simulink model "scdairframe_reference"  (Simulink 7.6)
settings: Solver=ode45  SolverMode=SingleTasking  StartTime=0.0  StopTime=10.0  RelTol=1e-3  AbsTol=1e-6
model workspace (MATLAB code in the model file):
  | scd_aero_guid_dat
values from neighbouring files (symbols this model uses):
  h_ini = 10000/m2ft    (= 3047.99990246)    [scd_aero_guid_dat.m]
  Thrust = 10e3    (= 10000)    [scd_aero_guid_dat.m]
libraries: aerospace x1
settings Model: Creator=The MathWorks Inc.  ExtModeTrigMode=oneshot  ExtModeArmWhenConnect=off  ExtModeAutoUpdateStatusClock=off
settings DataIOCC: LimitDataPoints=off  SaveOutput=off  SignalLogging=off  SaveTime=off  SignalLoggingName=sigsOut
settings OptimizationCC: BlockReduction=off  BooleanDataType=off  InlineParams=on  InlineInvariantSignals=on  InitFltsAndDblsToZero=on
settings DebuggingCC: SaveWithParameterizedLinksMsg=none  CheckExecutionContextPreStartOutputMsg=on  CheckExecutionContextRuntimeOutputMsg=on  SolverPrmCheckMsg=none  MultiTaskDSMMsg=warning  SigSpecEnsureSampleTimeMsg=none  StrictBusMsg=None
settings HardwareCC: TargetUnknown=on
settings GRTTargetCC: TargetFcnLib=ansi_tfl_tmw.mat

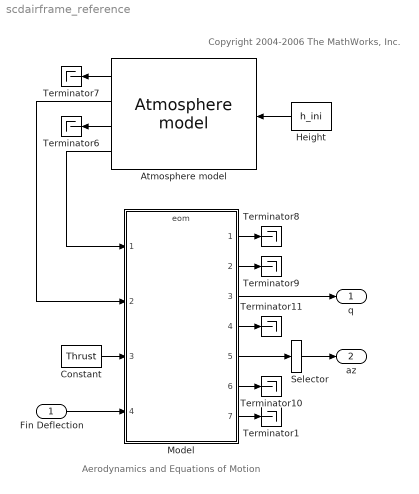
== system scdairframe_reference ==
  note: Aerodynamics and Equations of Motion
  note: Copyright 2004-2006 The MathWorks, Inc.
  Fin Deflection : Inport
  Atmosphere model : aerospace/Atmosphere/Atmosphere model  SystemSampleTime=-1
  Constant : Constant  Value=Thrust
  Height : Constant  Value=h_ini
  Model : ModelReference  ModelNameDialog=eom  SimulationMode=Accelerator  ModelReferenceVersion=1.8  CopyOfModelName=eom
  Selector : Selector  InputPortWidth=2  IndexOptions=Index vector (dialog)  Indices=[2]  OutputSizes=1
  Terminator{1,6..11} (7 alike) : Terminator
  q : Outport  InitialOutput=0
  az : Outport  Port=2  InitialOutput=0
  wires:
  Height/1 -> Atmosphere model/1
  Atmosphere model/1 -> Terminator7/1
  Atmosphere model/3 -> Terminator6/1
  Constant/1 -> Model/3
  Fin Deflection/1 -> Model/4
  Model/1 -> Terminator8/1
  Model/2 -> Terminator9/1
  Model/3 -> q/1
  Model/4 -> Terminator11/1
  Model/5 -> Selector/1
  Model/6 -> Terminator10/1
  Atmosphere model/4 -> Model/1
  Atmosphere model/2 -> Model/2
  Selector/1 -> az/1
  Model/7 -> Terminator1/1
